simulink model "sfcndemo_cppcount"  (Simulink 6.0)
settings: Solver=FixedStepDiscrete  StartTime=0.0  StopTime=9.9  FixedStep=1  RelTol=1e-3
PostLoadFcn:
  | sfcndemo_rtwcmd;
settings Model: Creator=The MathWorks Inc.  LastModifiedBy=batserve  ExtModeTrigMode=oneshot  ExtModeArmWhenConnect=off  ExtModeAutoUpdateStatusClock=off  ProdHWDeviceType=Specified
settings DataIOCC: LimitDataPoints=off  SignalLoggingName=logsOut
settings OptimizationCC: BlockReduction=off  BooleanDataType=off  LifeSpan=1
settings DebuggingCC: CheckExecutionContextPreStartOutputMsg=on  CheckExecutionContextRuntimeOutputMsg=on  SolverPrmCheckMsg=none
settings HardwareCC: ProdHWDeviceType=Specified
settings RTWCC: SystemTargetFile=ert.tlc  MakeCommand="make_rtw USER_INCLUDES=\"-I/devel/A/build/matlab/simulink/src\" USER_SRCS=\"/devel/A/build/matlab/simulink/src/sfun_cppcount_cpp.cpp\""  TemplateMakefile=ert_default_tmf  RetainRTWFile=on  ProcessScript=ert_make_rtw_hook
settings CodeAppCC: IgnoreCustomStorageClasses=off
settings ERTTargetCC: TargetFcnLib=ansi_tfl_tmw.mat  GenFloatMathFcnCalls=ANSI_C  GenerateSampleERTMain=on  MatFileLogging=on  SupportContinuousTime=on  SupportNonInlinedSFcns=on  RootIOFormat=Individual Arguments  ERTCustomFileTemplate=example_file_process.tlc  InitialValueSource=Model

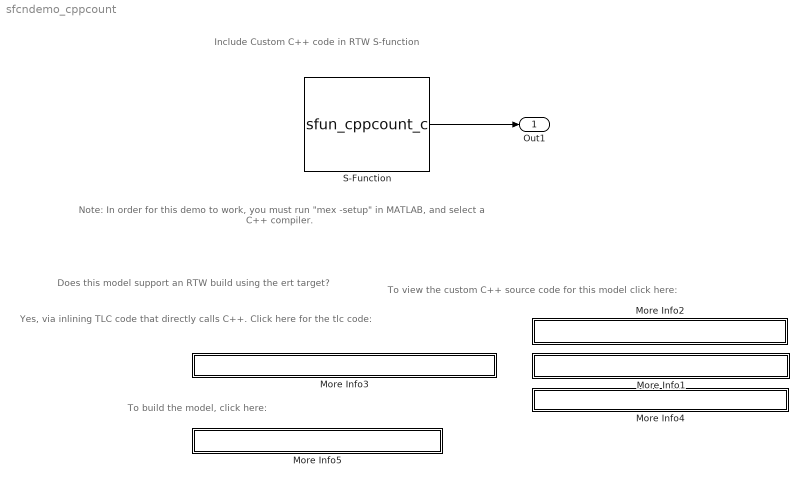
== system sfcndemo_cppcount ==
  note: To view the custom C++ source code for this model
      | click here:
  note: Does this model support an RTW build using
      | the ert target?
  note: Include Custom C++ code in RTW S-function
  note: Note: In order for this demo to work, you must run "mex -setup" in MATLAB, and
      | select a C++ compiler.
  note: Yes, via inlining TLC code that directly calls C++.
      | Click here for the tlc code:
  note: To build the model, click here:
  More Info1 : Subsystem  PropExecContextAcrossSSBoundary=on
      settings: OpenFcn=|
      | filename=fullfile(matlabroot, 'simulink', 'src', 'sfun_cppcount_c.c');
      | eval('edit(filename)')
      mask Display: disp('matlabroot\simulink\src\sfun_cppcount_c.c')
  More Info2 : Subsystem  PropExecContextAcrossSSBoundary=on
      settings: OpenFcn=|
      | filename=fullfile(matlabroot, 'simulink', 'src', 'sfun_cppcount_cpp.cpp');
      | eval('edit(filename)')
      mask Display: disp('matlabroot\simulink\src\sfun_cppcount_cpp.cpp')
  More Info3 : Subsystem  PropExecContextAcrossSSBoundary=on
      settings: OpenFcn=|
      | filename=fullfile(matlabroot, 'toolbox','simulink', 'blocks', 'tlc_c','sfun_cppcount_c.tlc');
      | eval('edit(filename)')
      mask Display: disp('matlabroot\toolbox\simulink\blocks\tlc_c\sfun_cppcount_c.tlc')
  More Info4 : Subsystem  PropExecContextAcrossSSBoundary=on
      settings: OpenFcn=|
      | filename=fullfile(matlabroot, 'simulink', 'src', 'sfun_cppcount_cpp.h');
      | eval('edit(filename)')
      mask Display: disp('matlabroot\simulink\src\sfun_cppcount_cpp.h')
  More Info5 : Subsystem  PropExecContextAcrossSSBoundary=on
      settings: OpenFcn=rtwbuild('sfcndemo_cppcount')
      mask Display: disp('Double click to build model with ERT target')
  S-Function : S-Function  FunctionName=sfun_cppcount_c  Parameters=1
  Out1 : Outport
  wires:
  S-Function/1 -> Out1/1

== system sfcndemo_cppcount/More Info1 ==

== system sfcndemo_cppcount/More Info2 ==

== system sfcndemo_cppcount/More Info3 ==

== system sfcndemo_cppcount/More Info4 ==

== system sfcndemo_cppcount/More Info5 ==
